simulink model "bd_par_auto2"  (Simulink 4.1.1)
settings: Solver=ode1  SolverMode=SingleTasking  StartTime=0.0  StopTime=max(cyc_mph(:,1))  FixedStep=1  MaxStep=1  RelTol=1e-3  AbsTol=1e-3
undefined symbols (not defined in the file): air_cp, amb_tmp, cs_charge_deplete_bool, cs_charge_trq, cs_electric_decel_spd, cs_electric_launch_spd_hi, cs_electric_launch_spd_lo, cs_hi_soc, cs_lo_soc, cs_min_trq_frac, cs_off_trq_frac, cyc_avg_time, cyc_cargo_mass, cyc_elevation_init, cyc_filter_bool, cyc_grade, cyc_mph, enable_stop, ess_cap_scale, ess_coulombic_eff, ess_init_soc, ess_max_ah_cap, ess_max_volts, ess_min_volts, ess_mod_airflow, ess_mod_cp, ess_mod_init_tmp, ess_module_mass, ess_module_num, ess_on, ess_res_scale_coef, ess_res_scale_fun, ess_set_tmp, ess_th_calc, ess_th_res_off, ess_th_res_on, ess_tmp, ess_voc, ex_calc, fc_ct_trq, fc_emis, fc_inertia, fc_map_spd, fc_max_trq, fc_on, fc_spd_scale, fc_trq_scale, fc_tstat, fd_inertia, fd_loss, fd_ratio, gb_dnshift_load, gb_dnshift_spd, gb_gears_num, gb_inertia, gb_num_init, gb_ratio, gb_shift_delay, gb_spd_scale, gb_trq_scale ... (+56)
libraries: lib_wheel2 x12, lib_accessory2 x3, lib_etc x2, lib_drive_cycle2 x1, lib_interactive x1, lib_drive_cycle x1, lib_exhaust x1, lib_fuel_converter3 x1
(part 14 of 18)

== system bd_par_auto2/motor/controller <mc>/motor model & interface/mc model/motor speed estimator ==
  mc_spd_out_a : Inport  Port=1  LatchInput=off
  <= max spd : Saturate  UpperLimit=max(mc_map_spd)*mc_spd_scale  LowerLimit=-inf  LinearizeAsGain=on
  Block NOTES : Subsystem
      settings: RTWFcnNameOpts=Auto  RTWFileNameOpts=Auto
      mask Display: disp('Block\nNOTES')
  Constant : Constant  Orientation=left  Value=eps
  Constant1 : Constant  Orientation=left  Value=0
  Constant2 : Constant  Orientation=left  Value=2
  Gain : Gain  Gain=0.447  Multiplication=Element-wise(K.*u)  SaturateOnIntegerOverflow=on
  IC : InitialCondition  Value=1
  Logical Operator1 : Logic  Operator=AND  Inputs=2
  Memory : Memory  Orientation=down  X0=0  InheritSampleTime=off
      settings: RTWStateStorageClass=Auto
  Memory2 : Memory  X0=0  InheritSampleTime=off
      settings: RTWStateStorageClass=Auto
  Product : Product  Inputs=**/  Multiplication=Element-wise(.*)  SaturateOnIntegerOverflow=on
  Relational : RelationalOperator  Operator=>
  Relational Operator1 : RelationalOperator  Operator=~=
  Sum : Sum  Inputs=++  SaturateOnIntegerOverflow=on
  Sum1 : Sum  Inputs=-+  SaturateOnIntegerOverflow=on
  Switch : Switch  Threshold=eps
  Switch1 : Switch  Threshold=eps
  enhancedToWorkspace : Subsystem  mask(enhancedToWorkspace){generalName=generalName, specificName=spd_est, logFlag=logFlag}
      mask prompts: generalName "General Name [char-evaluated]"; specificName "Specific Name [char-literal]"; logFlag "Enable flag (1=on,0=off)"
      mask help: A wrapper for the Simulink "To Workspace" block that allows you to evaluate the name of the variable to log to workspace. This is useful to avoid the double logging errors that occur when you pull in two library models that attempt to log to the same variable.
      mask init:
      | enhancedToWsMaker
      settings: CopyFcn=breakLinkCopyFcn  ParentCloseFcn=breakLinkParCloseFcn  RTWFcnNameOpts=Auto  RTWFileNameOpts=Auto
      mask Help:
      | <h2>Enhanced To Workspace Block</h2>
      | <h3>Parameters</h3>
      | <UL>
      | <li><b>General Name:</b> This is the more general name of the variable. Variables are saved to the workspace as <i>generalName_specificName</i>. Note that this is an evaluated variable. If you would like to type in the value directly, it must be surrounded with single quotes. Otherwise you can input the name of a variable containing a char string.</li>
      | <li><b>Specific Name:</b> This is the specific name of the variable. Note that this is input as a char literal (i.e., you don't need quotes).</li>
      | <li><b>Enable Flag:</b> This flag should have the value of 0 or 1. If 0, the variable will not be logged to the workspace. If 1, the variable will be logged. This is done so that variable logging can be turned off to improve speed.</li>
      | </ul>
      | <h3>Overview</h3>
      | <p>The enhanced to workspace block was put together to allow one to dynamically resolve variable names at run time in simulink. This is most powerful when used in conjunction with a masked subsystem to allow multiple instances of that masked subsytem to be used in the same model. The strategy is to set the generalName in the block mask which will allow the block to change the general name for all variable logging on the fly.
      | <h3>Helper Files</h3>
      | <p>Three m-files are required by the enhancedToWorkspace block. These files are located in the &lt; ADVISOR root &gt;/GUI directory :
      | <ul>
      | <li><i>enhancedToWsMaker.m</i> This file runs the mask initialization for the block</li>
      | <li><i>breakLinkCopyFcn.m</i> This file is used by the block callback when the simulink block is copied. It is necessary to break the link to the enhancedToWorkspace similar to the To Workspace block in order for it to be able to configure itself. (Try copying simulink's To Workspace block--it is impossible to make a link)</li>
      | <li><i>breakLinkParCloseFcn.m</i> This file is similar to the breakLinkCopyFcn and is used when a parent system is closed</li>
      | </ul>
      | <hr>
      | 
      | <p>Created 2003-Jan-21, Michael Patrick O'Keefe, NREL</p>
      mask Display: disp([generalName,'_',specificName])
  init via port : Subsystem
      settings: RTWFcnNameOpts=Auto  RTWFileNameOpts=Auto
  Out1 : Outport  Port=1
  tag scope: mc_spd_limited=scoped
  wires:
  Switch/1 -> init via port/1(signal in)
  IC/1 -> Switch1/2
  Relational/1 -> IC/1
  Sum1/1 -> Relational/1
  Constant2/1 -> Relational/2
  [mpha_prev] -> Sum1/1, Gain/1
  [cyc_mph_r_prev] -> Sum1/2
  Constant/1 -> Sum/2
  init via port/1(signal out) -> Switch1/1
  Constant1/1 -> Switch/3
  [veh_spd_a_rec_prev] -> Switch/2, Sum/1
  Gain/1 -> Product/2
  Sum/1 -> Product/3
  Product/1 -> Switch/1
  mc_spd_out_a/1 -> Switch1/3, Memory/1
  Memory2/1 -> Logical Operator1/2
  Logical Operator1/1 -> [mc_spd_limited]
  Relational Operator1/1 -> Logical Operator1/1, Memory2/1
  Switch1/1 -> <= max spd/1, Relational Operator1/1
  <= max spd/1 -> enhancedToWorkspace/1(In1), Out1/1, Relational Operator1/2
  [mc_init_spd_est] -> init via port/2(signal init)
  Memory/1 -> Product/1

== system bd_par_auto2/motor/controller <mc>/motor model & interface/mc model/rotor drive torque available (Nm) ==
  torque per unit input power (N-m/W) : Inport  Port=1  LatchInput=off
  available input power (W) : Inport  Port=2  LatchInput=off
  Block NOTES : Subsystem
      settings: RTWFcnNameOpts=Auto  RTWFileNameOpts=Auto
      mask Display: disp('Block\nNOTES')
  Constant2 : Constant  Value=inf
  Constant3 : Constant  Value=0
  Product : Product  Inputs=2  Multiplication=Element-wise(.*)  SaturateOnIntegerOverflow=on
  Relational Operator : RelationalOperator  Operator=~=
  Switch : Switch  Threshold=eps
  rotor drive torque available : Outport  Port=1  InitialOutput=0
  wires:
  torque per unit input power (N-m/W)/1 -> Relational Operator/1, Product/1
  Switch/1 -> rotor drive torque available/1
  Relational Operator/1 -> Switch/2
  Product/1 -> Switch/1
  available input power (W)/1 -> Product/2
  Constant2/1 -> Relational Operator/2
  Constant3/1 -> Switch/3

== system bd_par_auto2/power bus <pb>/power bus/model/Block NOTES ==
  note: This power bus requires power from (or distributes power to)
      | the generator first, taking the balance from the energy
      | storage system.

== system bd_par_auto2/power bus <pb>/power bus/model/enhancedToWorkspace ==
  In1 : Inport  Port=1  LatchInput=off
  To Workspace : ToWorkspace  VariableName=pb_pwr_out_r  SampleTime=-1  SaveFormat=Array
  wires:
  In1/1 -> To Workspace/1

== system bd_par_auto2/power bus <pb>/power bus/model/enhancedToWorkspace1 ==
  In1 : Inport  Port=1  LatchInput=off
  To Workspace : ToWorkspace  VariableName=pb_pwr_out_a  SampleTime=-1  SaveFormat=Array
  wires:
  In1/1 -> To Workspace/1

== system bd_par_auto2/torque coupler <tc>/tc model & interface/tc model/Block NOTES ==
  note: speed, while the motor's speed may be different.  The ratio of motor speed to main
      | output speed is stored in the variable tc_mc_to_fc_spd_ratio.
  note: This block models a chain- or belt-driven torque coupler, with three gears:  one each
      | for the motor, main input (the engine or gearbox), and main output (to the gearbox
      | or final drive).  It includes losses in the chain or belt, but leaves inertia effects to be
      | considered in the appropriate component.
      |
      | The entire torque required out of the torque coupler (plus losses) is required from the
      | engine.  The engine provides only as much torque as its engine controller (see the
      | <vc> block) allows.  Any remaining unmet torque request is submitted to the motor,
      | which meets the request to the best of its ability.
      |
      | The torque converter output speed is limited by the maximum speeds of both the
      | motor and the engine.
      |
      | The loss torque is zero when the gears are not turning, and is applied at the output
      |  gear.
      |
      | The gears connecting the main input and main output to the torque converter's belt
      | or chain are assumed to be of the same size, so that main input speed = main output

== system bd_par_auto2/torque coupler <tc>/tc model & interface/tc model/enhancedToWorkspace ==
  In1 : Inport  Port=1  LatchInput=off
  Terminator : Terminator
  wires:
  In1/1 -> Terminator/1

== system bd_par_auto2/torque coupler <tc>/tc model & interface/tc model/enhancedToWorkspace1 ==
  In1 : Inport  Port=1  LatchInput=off
  Terminator : Terminator
  wires:
  In1/1 -> Terminator/1

== system bd_par_auto2/torque coupler <tc>/tc model & interface/tc model/enhancedToWorkspace2 ==
  In1 : Inport  Port=1  LatchInput=off
  Terminator : Terminator
  wires:
  In1/1 -> Terminator/1

== system bd_par_auto2/torque coupler <tc>/tc model & interface/tc model/enhancedToWorkspace3 ==
  In1 : Inport  Port=1  LatchInput=off
  Terminator : Terminator
  wires:
  In1/1 -> Terminator/1

== system bd_par_auto2/torque coupler <tc>/tc model & interface/tc model/enhancedToWorkspace4 ==
  In1 : Inport  Port=1  LatchInput=off
  Terminator : Terminator
  wires:
  In1/1 -> Terminator/1

== system bd_par_auto2/torque coupler <tc>/tc model & interface/tc model/help ==

== system bd_par_auto2/torque coupler <tc>/tc model & interface/tc model/loss (Nm) ==
  note: The loss torque is zero when the gears are not turning,
      | and is applied at the torque coupler's output gear.
  tc output speed (rad/s) : Inport  Port=1  LatchInput=off
  Constant : Constant  Orientation=up  Value=0
  Switch : Switch  Threshold=eps
  torque coupler loss torque (Nm) : Constant  Value=tc_loss
  drag torque (Nm) : Outport  Port=1  InitialOutput=0
  wires:
  torque coupler loss torque (Nm)/1 -> Switch/1
  Switch/1 -> drag torque (Nm)/1
  tc output speed (rad/s)/1 -> Switch/2
  Constant/1 -> Switch/3

== system bd_par_auto2/torque modification  strategy <cs>/torque mod  model & interface/model/help ==

== system bd_par_auto2/vehicle, wheel, & axle front/rear <wh> 2 axle --> 1 driveline/models and interface/vehicle <veh>/Block NOTES ==
  note: 2003-April-02, Michael O'Keefe
      | Model updated to use a "stand-alone" mask format
  note: A slight simplification, the assumption that (speed_at_end_of_time_step)^2 is roughly equal to
      | (speed_at_end_of_time_step)*(speed_at_beginning_of_time_step), is used to avoid solving
      | a quadratic equation in the solution of v=v(Ftract).
  note: This block uses the required vehicle speed with vehicle parameters and the previous speed
      | and classic, straightforward equations to determine the tractive force required at the tire/road interface.
  note: If no drivetrain component ran up against its performance limit during the time step, the achieved speed
      | is taken to be the requested speed.
  note: Given the tractive force available, this block uses the same equations to determine the achievable speed.

== system bd_par_auto2/vehicle, wheel, & axle front/rear <wh> 2 axle --> 1 driveline/models and interface/vehicle <veh>/enhancedToWorkspace ==
  In1 : Inport  Port=1  LatchInput=off
  To Workspace : ToWorkspace  VariableName=veh_spd_a  SampleTime=-1  SaveFormat=Array
  wires:
  In1/1 -> To Workspace/1

== system bd_par_auto2/vehicle, wheel, & axle front/rear <wh> 2 axle --> 1 driveline/models and interface/vehicle <veh>/enhancedToWorkspace1 ==
  In1 : Inport  Port=1  LatchInput=off
  To Workspace : ToWorkspace  VariableName=veh_force_a  SampleTime=-1  SaveFormat=Array
  wires:
  In1/1 -> To Workspace/1

== system bd_par_auto2/vehicle, wheel, & axle front/rear <wh> 2 axle --> 1 driveline/models and interface/vehicle <veh>/enhancedToWorkspace2 ==
  In1 : Inport  Port=1  LatchInput=off
  To Workspace : ToWorkspace  VariableName=veh_spd_r  SampleTime=-1  SaveFormat=Array
  wires:
  In1/1 -> To Workspace/1

== system bd_par_auto2/vehicle, wheel, & axle front/rear <wh> 2 axle --> 1 driveline/models and interface/vehicle <veh>/enhancedToWorkspace3 ==
  In1 : Inport  Port=1  LatchInput=off
  To Workspace : ToWorkspace  VariableName=veh_force_r  SampleTime=-1  SaveFormat=Array
  wires:
  In1/1 -> To Workspace/1

== system bd_par_auto2/vehicle, wheel, & axle front/rear <wh> 2 axle --> 1 driveline/models and interface/vehicle <veh>/enhancedToWorkspace4 ==
  In1 : Inport  Port=1  LatchInput=off
  To Workspace : ToWorkspace  VariableName=veh_Fr  SampleTime=-1  SaveFormat=Array
  wires:
  In1/1 -> To Workspace/1

== system bd_par_auto2/vehicle, wheel, & axle front/rear <wh> 2 axle --> 1 driveline/models and interface/vehicle <veh>/force req'd to accelerate (N) ==
  v(m/s) : Inport  Port=1  LatchInput=off
  v prev : Inport  Port=2  LatchInput=off
  Clock : Clock
      settings: DisplayTime=off  Decimation=10
  Memory : Memory  X0=-0.1  InheritSampleTime=off
      settings: RTWStateStorageClass=Auto
  Product1 : Product  Inputs=**/  Multiplication=Element-wise(.*)  SaturateOnIntegerOverflow=on
  Sum : Sum  Inputs=+-  SaturateOnIntegerOverflow=on
  Sum1 : Sum  Inputs=+-  SaturateOnIntegerOverflow=on
  current veh mass : lib_wheel2/Submodels/current veh mass
      settings: RTWFcnNameOpts=Auto  RTWFileNameOpts=Auto
  (N) : Outport  Port=1  InitialOutput=0
  wires:
  current veh mass/1 -> Product1/1
  Clock/1 -> Sum1/1, Memory/1
  Memory/1 -> Sum1/2
  Product1/1 -> (N)/1
  v prev/1 -> Sum/2
  v(m/s)/1 -> Sum/1
  Sum1/1 -> Product1/3
  Sum/1 -> Product1/2

== system bd_par_auto2/vehicle, wheel, & axle front/rear <wh> 2 axle --> 1 driveline/models and interface/vehicle <veh>/force req'd to ascend (N) ==
  average vehicle speed over time step (m/s) : Inport  Port=1  LatchInput=off
  Constant : Constant  Value=veh_gravity
  Constant1 : Constant  Value=0
  Product : Product  Inputs=3  Multiplication=Element-wise(.*)  SaturateOnIntegerOverflow=on
  Switch : Switch  Threshold=0
  Trigonometric Function : Trigonometry  Operator=atan  OutputSignalType=auto
  Trigonometric Function1 : Trigonometry  Operator=sin  OutputSignalType=auto
  current veh mass : lib_wheel2/Submodels/current veh mass
      settings: RTWFcnNameOpts=Auto  RTWFileNameOpts=Auto
  (N) : Outport  Port=1  InitialOutput=0
  wires:
  current veh mass/1 -> Product/3
  average vehicle speed over time step (m/s)/1 -> Switch/2
  Constant1/1 -> Switch/3
  Switch/1 -> (N)/1
  Product/1 -> Switch/1
  Constant/1 -> Product/1
  [grade] -> Trigonometric Function/1
  Trigonometric Function1/1 -> Product/2
  Trigonometric Function/1 -> Trigonometric Function1/1

== system bd_par_auto2/vehicle, wheel, & axle front/rear <wh> 2 axle --> 1 driveline/models and interface/vehicle <veh>/force req'd to overcome aerodynamic drag (N) ==
  average vehicle speed over time step (m/s) : Inport  Port=1  LatchInput=off
  Constant : Constant  Value=veh_air_density*veh_CD*veh_FA*0.5
  Product : Product  Inputs=3  Multiplication=Element-wise(.*)  SaturateOnIntegerOverflow=on
  D aero(N) : Outport  Port=1  InitialOutput=0
  wires:
  Product/1 -> D aero(N)/1
  Constant/1 -> Product/3
  average vehicle speed over time step (m/s)/1 -> Product/2, Product/1

== system bd_par_auto2/vehicle, wheel, & axle front/rear <wh> 2 axle --> 1 driveline/models and interface/vehicle <veh>/help ==

== system bd_par_auto2/vehicle, wheel, & axle front/rear <wh> 2 axle --> 1 driveline/models and interface/vehicle <veh>/memory & init speed ==
  note: 2003-April-02, Michael O'Keefe
      |
      | This block passes through the last speed achieved unless this is the initial condition in which
      | case the initial speed value (a supplied control signal) is passed through. For backwards
      | compatibility, the value of v_init should be cyc_mph(1,2)*0.447
  note: cyc_mph(1,2)*.447
  signal in : Inport  Port=1  LatchInput=off
  signal init : Inport  Port=2  LatchInput=off
  Constant : Constant  Value=1
  IC : InitialCondition  Value=0
  Memory : Memory  X0=0  InheritSampleTime=off
      settings: RTWStateStorageClass=Auto
  Switch : Switch  Threshold=0.5
  signal out : Outport  Port=1
  wires:
  signal init/1 -> Switch/3
  Switch/1 -> signal out/1
  IC/1 -> Switch/2
  Memory/1 -> Switch/1
  Constant/1 -> IC/1
  signal in/1 -> Memory/1

== system bd_par_auto2/vehicle, wheel, & axle front/rear <wh> 2 axle --> 1 driveline/models and interface/vehicle <veh>/power logging--achieved ==
  veh_force_a : Inport  Port=1  LatchInput=off
  veh_spd_a : Inport  Port=2  LatchInput=off
  Integrator : Integrator  ExternalReset=none  InitialConditionSource=internal  InitialCondition=0  LimitOutput=off  UpperSaturationLimit=inf  LowerSaturationLimit=-inf  ShowSaturationPort=off  ShowStatePort=off  AbsoluteTolerance=auto
  Joules : Subsystem  TreatAsAtomicUnit=on  mask(enhancedToWorkspace){generalName=generalName, specificName=energy_a, logFlag=logFlag}
      mask prompts: generalName "General Name [char-evaluated]"; specificName "Specific Name [char-literal]"; logFlag "Enable flag (1=on,0=off)"
      mask help: A wrapper for the Simulink "To Workspace" block that allows you to evaluate the name of the variable to log to workspace. This is useful to avoid the double logging errors that occur when you pull in two library models that attempt to log to the same variable.
      mask init:
      | enhancedToWsMaker
      settings: CopyFcn=breakLinkCopyFcn  ParentCloseFcn=breakLinkParCloseFcn  RTWFcnNameOpts=Auto  RTWFileNameOpts=Auto
      mask Help:
      | <h2>Enhanced To Workspace Block</h2>
      | <h3>Parameters</h3>
      | <UL>
      | <li><b>General Name:</b> This is the more general name of the variable. Variables are saved to the workspace as <i>generalName_specificName</i>. Note that this is an evaluated variable. If you would like to type in the value directly, it must be surrounded with single quotes. Otherwise you can input the name of a variable containing a char string.</li>
      | <li><b>Specific Name:</b> This is the specific name of the variable. Note that this is input as a char literal (i.e., you don't need quotes).</li>
      | <li><b>Enable Flag:</b> This flag should have the value of 0 or 1. If 0, the variable will not be logged to the workspace. If 1, the variable will be logged. This is done so that variable logging can be turned off to improve speed.</li>
      | </ul>
      | <h3>Overview</h3>
      | <p>The enhanced to workspace block was put together to allow one to dynamically resolve variable names at run time in simulink. This is most powerful when used in conjunction with a masked subsystem to allow multiple instances of that masked subsytem to be used in the same model. The strategy is to set the generalName in the block mask which will allow the block to change the general name for all variable logging on the fly.
      | <h3>Helper Files</h3>
      | <p>Three m-files are required by the enhancedToWorkspace block. These files are located in the &lt; ADVISOR root &gt;/GUI directory :
      | <ul>
      | <li><i>enhancedToWsMaker.m</i> This file runs the mask initialization for the block</li>
      | <li><i>breakLinkCopyFcn.m</i> This file is used by the block callback when the simulink block is copied. It is necessary to break the link to the enhancedToWorkspace similar to the To Workspace block in order for it to be able to configure itself. (Try copying simulink's To Workspace block--it is impossible to make a link)</li>
      | <li><i>breakLinkParCloseFcn.m</i> This file is similar to the breakLinkCopyFcn and is used when a parent system is closed</li>
      | </ul>
      | <hr>
      | 
      | <p>Created 2003-Jan-21, Michael Patrick O'Keefe, NREL</p>
      | 
      | <!--
      | <VARDEF>
      | <H3>var_name</H3>
      | <UL>
      | <LI><B>data type</B> data type here</LI>
      | <LI><B>units</B> units here</LI>
      | <LI><B>vehicle type</B> vehicle type here</LI>
      | <LI><B>description</B> description here</LI>
      | </UL>
      | </VARDEF>
      | -->
      mask Display: disp([generalName,'_',specificName])
  Product : Product  Inputs=2  Multiplication=Element-wise(.*)  SaturateOnIntegerOverflow=on
  horse power : Subsystem  TreatAsAtomicUnit=on  mask(enhancedToWorkspace){generalName=generalName, specificName=pwr_a_hp, logFlag=logFlag}
      mask prompts: generalName "General Name [char-evaluated]"; specificName "Specific Name [char-literal]"; logFlag "Enable flag (1=on,0=off)"
      mask help: A wrapper for the Simulink "To Workspace" block that allows you to evaluate the name of the variable to log to workspace. This is useful to avoid the double logging errors that occur when you pull in two library models that attempt to log to the same variable.
      mask init:
      | enhancedToWsMaker
      settings: CopyFcn=breakLinkCopyFcn  ParentCloseFcn=breakLinkParCloseFcn  RTWFcnNameOpts=Auto  RTWFileNameOpts=Auto
      mask Help:
      | <h2>Enhanced To Workspace Block</h2>
      | <h3>Parameters</h3>
      | <UL>
      | <li><b>General Name:</b> This is the more general name of the variable. Variables are saved to the workspace as <i>generalName_specificName</i>. Note that this is an evaluated variable. If you would like to type in the value directly, it must be surrounded with single quotes. Otherwise you can input the name of a variable containing a char string.</li>
      | <li><b>Specific Name:</b> This is the specific name of the variable. Note that this is input as a char literal (i.e., you don't need quotes).</li>
      | <li><b>Enable Flag:</b> This flag should have the value of 0 or 1. If 0, the variable will not be logged to the workspace. If 1, the variable will be logged. This is done so that variable logging can be turned off to improve speed.</li>
      | </ul>
      | <h3>Overview</h3>
      | <p>The enhanced to workspace block was put together to allow one to dynamically resolve variable names at run time in simulink. This is most powerful when used in conjunction with a masked subsystem to allow multiple instances of that masked subsytem to be used in the same model. The strategy is to set the generalName in the block mask which will allow the block to change the general name for all variable logging on the fly.
      | <h3>Helper Files</h3>
      | <p>Three m-files are required by the enhancedToWorkspace block. These files are located in the &lt; ADVISOR root &gt;/GUI directory :
      | <ul>
      | <li><i>enhancedToWsMaker.m</i> This file runs the mask initialization for the block</li>
      | <li><i>breakLinkCopyFcn.m</i> This file is used by the block callback when the simulink block is copied. It is necessary to break the link to the enhancedToWorkspace similar to the To Workspace block in order for it to be able to configure itself. (Try copying simulink's To Workspace block--it is impossible to make a link)</li>
      | <li><i>breakLinkParCloseFcn.m</i> This file is similar to the breakLinkCopyFcn and is used when a parent system is closed</li>
      | </ul>
      | <hr>
      | 
      | <p>Created 2003-Jan-21, Michael Patrick O'Keefe, NREL</p>
      | 
      | <!--
      | <VARDEF>
      | <H3>var_name</H3>
      | <UL>
      | <LI><B>data type</B> data type here</LI>
      | <LI><B>units</B> units here</LI>
      | <LI><B>vehicle type</B> vehicle type here</LI>
      | <LI><B>description</B> description here</LI>
      | </UL>
      | </VARDEF>
      | -->
      mask Display: disp([generalName,'_',specificName])
  "w -> hp" : Gain  Gain=0.001341022  Multiplication=Element-wise(K.*u)  SaturateOnIntegerOverflow=on
  watts : Subsystem  TreatAsAtomicUnit=on  mask(enhancedToWorkspace){generalName=generalName, specificName=pwr_a, logFlag=logFlag}
      mask prompts: generalName "General Name [char-evaluated]"; specificName "Specific Name [char-literal]"; logFlag "Enable flag (1=on,0=off)"
      mask help: A wrapper for the Simulink "To Workspace" block that allows you to evaluate the name of the variable to log to workspace. This is useful to avoid the double logging errors that occur when you pull in two library models that attempt to log to the same variable.
      mask init:
      | enhancedToWsMaker
      settings: CopyFcn=breakLinkCopyFcn  ParentCloseFcn=breakLinkParCloseFcn  RTWFcnNameOpts=Auto  RTWFileNameOpts=Auto
      mask Help:
      | <h2>Enhanced To Workspace Block</h2>
      | <h3>Parameters</h3>
      | <UL>
      | <li><b>General Name:</b> This is the more general name of the variable. Variables are saved to the workspace as <i>generalName_specificName</i>. Note that this is an evaluated variable. If you would like to type in the value directly, it must be surrounded with single quotes. Otherwise you can input the name of a variable containing a char string.</li>
      | <li><b>Specific Name:</b> This is the specific name of the variable. Note that this is input as a char literal (i.e., you don't need quotes).</li>
      | <li><b>Enable Flag:</b> This flag should have the value of 0 or 1. If 0, the variable will not be logged to the workspace. If 1, the variable will be logged. This is done so that variable logging can be turned off to improve speed.</li>
      | </ul>
      | <h3>Overview</h3>
      | <p>The enhanced to workspace block was put together to allow one to dynamically resolve variable names at run time in simulink. This is most powerful when used in conjunction with a masked subsystem to allow multiple instances of that masked subsytem to be used in the same model. The strategy is to set the generalName in the block mask which will allow the block to change the general name for all variable logging on the fly.
      | <h3>Helper Files</h3>
      | <p>Three m-files are required by the enhancedToWorkspace block. These files are located in the &lt; ADVISOR root &gt;/GUI directory :
      | <ul>
      | <li><i>enhancedToWsMaker.m</i> This file runs the mask initialization for the block</li>
      | <li><i>breakLinkCopyFcn.m</i> This file is used by the block callback when the simulink block is copied. It is necessary to break the link to the enhancedToWorkspace similar to the To Workspace block in order for it to be able to configure itself. (Try copying simulink's To Workspace block--it is impossible to make a link)</li>
      | <li><i>breakLinkParCloseFcn.m</i> This file is similar to the breakLinkCopyFcn and is used when a parent system is closed</li>
      | </ul>
      | <hr>
      | 
      | <p>Created 2003-Jan-21, Michael Patrick O'Keefe, NREL</p>
      | 
      | <!--
      | <VARDEF>
      | <H3>var_name</H3>
      | <UL>
      | <LI><B>data type</B> data type here</LI>
      | <LI><B>units</B> units here</LI>
      | <LI><B>vehicle type</B> vehicle type here</LI>
      | <LI><B>description</B> description here</LI>
      | </UL>
      | </VARDEF>
      | -->
      mask Display: disp([generalName,'_',specificName])
  wires:
  "w -> hp"/1 -> horse power/1(In1)
  Product/1 -> "w -> hp"/1, Integrator/1, watts/1(In1)
  Integrator/1 -> Joules/1(In1)
  veh_force_a/1 -> Product/1
  veh_spd_a/1 -> Product/2

== system bd_par_auto2/vehicle, wheel, & axle front/rear <wh> 2 axle --> 1 driveline/models and interface/vehicle <veh>/power logging--request ==
  veh_force_r : Inport  Port=1  LatchInput=off
  veh_spd_r : Inport  Port=2  LatchInput=off
  Integrator : Integrator  ExternalReset=none  InitialConditionSource=internal  InitialCondition=0  LimitOutput=off  UpperSaturationLimit=inf  LowerSaturationLimit=-inf  ShowSaturationPort=off  ShowStatePort=off  AbsoluteTolerance=auto
  Joules : Subsystem  TreatAsAtomicUnit=on  mask(enhancedToWorkspace){generalName=generalName, specificName=energy_r, logFlag=logFlag}
      mask prompts: generalName "General Name [char-evaluated]"; specificName "Specific Name [char-literal]"; logFlag "Enable flag (1=on,0=off)"
      mask help: A wrapper for the Simulink "To Workspace" block that allows you to evaluate the name of the variable to log to workspace. This is useful to avoid the double logging errors that occur when you pull in two library models that attempt to log to the same variable.
      mask init:
      | enhancedToWsMaker
      settings: CopyFcn=breakLinkCopyFcn  ParentCloseFcn=breakLinkParCloseFcn  RTWFcnNameOpts=Auto  RTWFileNameOpts=Auto
      mask Help:
      | <h2>Enhanced To Workspace Block</h2>
      | <h3>Parameters</h3>
      | <UL>
      | <li><b>General Name:</b> This is the more general name of the variable. Variables are saved to the workspace as <i>generalName_specificName</i>. Note that this is an evaluated variable. If you would like to type in the value directly, it must be surrounded with single quotes. Otherwise you can input the name of a variable containing a char string.</li>
      | <li><b>Specific Name:</b> This is the specific name of the variable. Note that this is input as a char literal (i.e., you don't need quotes).</li>
      | <li><b>Enable Flag:</b> This flag should have the value of 0 or 1. If 0, the variable will not be logged to the workspace. If 1, the variable will be logged. This is done so that variable logging can be turned off to improve speed.</li>
      | </ul>
      | <h3>Overview</h3>
      | <p>The enhanced to workspace block was put together to allow one to dynamically resolve variable names at run time in simulink. This is most powerful when used in conjunction with a masked subsystem to allow multiple instances of that masked subsytem to be used in the same model. The strategy is to set the generalName in the block mask which will allow the block to change the general name for all variable logging on the fly.
      | <h3>Helper Files</h3>
      | <p>Three m-files are required by the enhancedToWorkspace block. These files are located in the &lt; ADVISOR root &gt;/GUI directory :
      | <ul>
      | <li><i>enhancedToWsMaker.m</i> This file runs the mask initialization for the block</li>
      | <li><i>breakLinkCopyFcn.m</i> This file is used by the block callback when the simulink block is copied. It is necessary to break the link to the enhancedToWorkspace similar to the To Workspace block in order for it to be able to configure itself. (Try copying simulink's To Workspace block--it is impossible to make a link)</li>
      | <li><i>breakLinkParCloseFcn.m</i> This file is similar to the breakLinkCopyFcn and is used when a parent system is closed</li>
      | </ul>
      | <hr>
      | 
      | <p>Created 2003-Jan-21, Michael Patrick O'Keefe, NREL</p>
      | 
      | <!--
      | <VARDEF>
      | <H3>var_name</H3>
      | <UL>
      | <LI><B>data type</B> data type here</LI>
      | <LI><B>units</B> units here</LI>
      | <LI><B>vehicle type</B> vehicle type here</LI>
      | <LI><B>description</B> description here</LI>
      | </UL>
      | </VARDEF>
      | -->
      mask Display: disp([generalName,'_',specificName])
  Product : Product  Inputs=2  Multiplication=Element-wise(.*)  SaturateOnIntegerOverflow=on
  horse power : Subsystem  TreatAsAtomicUnit=on  mask(enhancedToWorkspace){generalName=generalName, specificName=pwr_r_hp, logFlag=logFlag}
      mask prompts: generalName "General Name [char-evaluated]"; specificName "Specific Name [char-literal]"; logFlag "Enable flag (1=on,0=off)"
      mask help: A wrapper for the Simulink "To Workspace" block that allows you to evaluate the name of the variable to log to workspace. This is useful to avoid the double logging errors that occur when you pull in two library models that attempt to log to the same variable.
      mask init:
      | enhancedToWsMaker
      settings: CopyFcn=breakLinkCopyFcn  ParentCloseFcn=breakLinkParCloseFcn  RTWFcnNameOpts=Auto  RTWFileNameOpts=Auto
      mask Help:
      | <h2>Enhanced To Workspace Block</h2>
      | <h3>Parameters</h3>
      | <UL>
      | <li><b>General Name:</b> This is the more general name of the variable. Variables are saved to the workspace as <i>generalName_specificName</i>. Note that this is an evaluated variable. If you would like to type in the value directly, it must be surrounded with single quotes. Otherwise you can input the name of a variable containing a char string.</li>
      | <li><b>Specific Name:</b> This is the specific name of the variable. Note that this is input as a char literal (i.e., you don't need quotes).</li>
      | <li><b>Enable Flag:</b> This flag should have the value of 0 or 1. If 0, the variable will not be logged to the workspace. If 1, the variable will be logged. This is done so that variable logging can be turned off to improve speed.</li>
      | </ul>
      | <h3>Overview</h3>
      | <p>The enhanced to workspace block was put together to allow one to dynamically resolve variable names at run time in simulink. This is most powerful when used in conjunction with a masked subsystem to allow multiple instances of that masked subsytem to be used in the same model. The strategy is to set the generalName in the block mask which will allow the block to change the general name for all variable logging on the fly.
      | <h3>Helper Files</h3>
      | <p>Three m-files are required by the enhancedToWorkspace block. These files are located in the &lt; ADVISOR root &gt;/GUI directory :
      | <ul>
      | <li><i>enhancedToWsMaker.m</i> This file runs the mask initialization for the block</li>
      | <li><i>breakLinkCopyFcn.m</i> This file is used by the block callback when the simulink block is copied. It is necessary to break the link to the enhancedToWorkspace similar to the To Workspace block in order for it to be able to configure itself. (Try copying simulink's To Workspace block--it is impossible to make a link)</li>
      | <li><i>breakLinkParCloseFcn.m</i> This file is similar to the breakLinkCopyFcn and is used when a parent system is closed</li>
      | </ul>
      | <hr>
      | 
      | <p>Created 2003-Jan-21, Michael Patrick O'Keefe, NREL</p>
      | 
      | <!--
      | <VARDEF>
      | <H3>var_name</H3>
      | <UL>
      | <LI><B>data type</B> data type here</LI>
      | <LI><B>units</B> units here</LI>
      | <LI><B>vehicle type</B> vehicle type here</LI>
      | <LI><B>description</B> description here</LI>
      | </UL>
      | </VARDEF>
      | -->
      mask Display: disp([generalName,'_',specificName])
  "w -> hp" : Gain  Gain=0.001341022  Multiplication=Element-wise(K.*u)  SaturateOnIntegerOverflow=on
  watts : Subsystem  TreatAsAtomicUnit=on  mask(enhancedToWorkspace){generalName=generalName, specificName=pwr_r, logFlag=logFlag}
      mask prompts: generalName "General Name [char-evaluated]"; specificName "Specific Name [char-literal]"; logFlag "Enable flag (1=on,0=off)"
      mask help: A wrapper for the Simulink "To Workspace" block that allows you to evaluate the name of the variable to log to workspace. This is useful to avoid the double logging errors that occur when you pull in two library models that attempt to log to the same variable.
      mask init:
      | enhancedToWsMaker
      settings: CopyFcn=breakLinkCopyFcn  ParentCloseFcn=breakLinkParCloseFcn  RTWFcnNameOpts=Auto  RTWFileNameOpts=Auto
      mask Help:
      | <h2>Enhanced To Workspace Block</h2>
      | <h3>Parameters</h3>
      | <UL>
      | <li><b>General Name:</b> This is the more general name of the variable. Variables are saved to the workspace as <i>generalName_specificName</i>. Note that this is an evaluated variable. If you would like to type in the value directly, it must be surrounded with single quotes. Otherwise you can input the name of a variable containing a char string.</li>
      | <li><b>Specific Name:</b> This is the specific name of the variable. Note that this is input as a char literal (i.e., you don't need quotes).</li>
      | <li><b>Enable Flag:</b> This flag should have the value of 0 or 1. If 0, the variable will not be logged to the workspace. If 1, the variable will be logged. This is done so that variable logging can be turned off to improve speed.</li>
      | </ul>
      | <h3>Overview</h3>
      | <p>The enhanced to workspace block was put together to allow one to dynamically resolve variable names at run time in simulink. This is most powerful when used in conjunction with a masked subsystem to allow multiple instances of that masked subsytem to be used in the same model. The strategy is to set the generalName in the block mask which will allow the block to change the general name for all variable logging on the fly.
      | <h3>Helper Files</h3>
      | <p>Three m-files are required by the enhancedToWorkspace block. These files are located in the &lt; ADVISOR root &gt;/GUI directory :
      | <ul>
      | <li><i>enhancedToWsMaker.m</i> This file runs the mask initialization for the block</li>
      | <li><i>breakLinkCopyFcn.m</i> This file is used by the block callback when the simulink block is copied. It is necessary to break the link to the enhancedToWorkspace similar to the To Workspace block in order for it to be able to configure itself. (Try copying simulink's To Workspace block--it is impossible to make a link)</li>
      | <li><i>breakLinkParCloseFcn.m</i> This file is similar to the breakLinkCopyFcn and is used when a parent system is closed</li>
      | </ul>
      | <hr>
      | 
      | <p>Created 2003-Jan-21, Michael Patrick O'Keefe, NREL</p>
      | 
      | <!--
      | <VARDEF>
      | <H3>var_name</H3>
      | <UL>
      | <LI><B>data type</B> data type here</LI>
      | <LI><B>units</B> units here</LI>
      | <LI><B>vehicle type</B> vehicle type here</LI>
      | <LI><B>description</B> description here</LI>
      | </UL>
      | </VARDEF>
      | -->
      mask Display: disp([generalName,'_',specificName])
  wires:
  "w -> hp"/1 -> horse power/1(In1)
  Product/1 -> "w -> hp"/1, Integrator/1, watts/1(In1)
  Integrator/1 -> Joules/1(In1)
  veh_force_r/1 -> Product/1
  veh_spd_r/1 -> Product/2
